simulink model "untitled"  (R2018b)
settings: Solver=VariableStepAuto  StartTime=0.0  StopTime=50.0  RelTol=1e-3
values from neighbouring files (symbols this model uses):
  k1 = 0.6    [Regulation_temperature.m]
  k2 = -0.25    [Regulation_temperature.m]
libraries: cstblocks x2
settings Model: Creator=damatheu  LastModifiedBy=damatheu

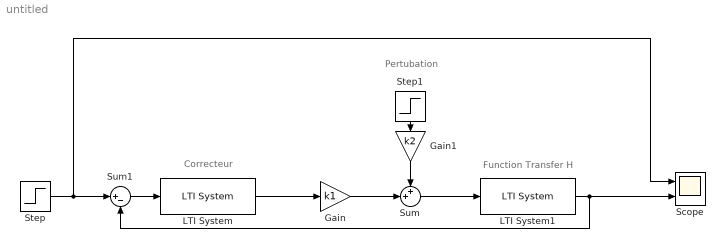
== system untitled ==
  note: Function Transfer H
  note: Correcteur
  note: Pertubation
  Gain : Gain  Gain=k1
  Gain1 : Gain  Gain=k2
  LTI System : cstblocks/LTI System  sys=C  IC=[]
  LTI System1 : cstblocks/LTI System  sys=H  IC=[]
  Scope : Scope  NumInputPorts=2
  Step : Step  SampleTime=0
  Step1 : Step  Time=2  SampleTime=0
  Sum : Sum  Inputs=++|
  Sum1 : Sum  Inputs=|+-
  wires:
  Step1/1 -> Gain1/1
  Gain1/1 -> Sum/1
  Gain/1 -> Sum/2
  LTI System/1 -> Gain/1
  Step/1 -> Scope/1, Sum1/1
  Sum/1 -> LTI System1/1
  LTI System1/1 -> Scope/2, Sum1/2
  Sum1/1 -> LTI System/1
